simulink model "slb_gain"  (R2015b)
settings: Solver=FixedStepDiscrete  SolverMode=SingleTasking  StartTime=0.0  StopTime=10.0  RelTol=1e-3
PreLoadFcn:
  | A1 = 4
  | A2 = 10
  | A3 = 231
libraries: simulink x3
settings Model: Creator=amatsumo  LastModifiedBy=amatsumo
settings DataIOCC: SaveFormat=Array  SignalLoggingSaveFormat=ModelDataLogs  SaveOutput=off  SignalLogging=off  SaveTime=off
settings OptimizationCC: BlockReduction=off  ConditionallyExecuteInputs=off  DefaultParameterBehavior=Inlined  ExpressionDepthLimit=2147483647
settings DebuggingCC: AlgebraicLoopMsg=error  UnderspecifiedInitializationDetection=Classic  MergeDetectMultiDrivingBlocksExec=none  SolverPrmCheckMsg=warning  InheritedTsInSrcMsg=none  SingleTaskRateTransMsg=error  FcnCallInpInsideContextMsg=UseLocalSettings  StateNameClashWarn=warning
settings HardwareCC: ProdBitPerPointer=32  ProdLargestAtomicFloat=None  ProdIntDivRoundTo=Undefined  ProdEndianess=Unspecified  ProdWordSize=32  ProdHWDeviceType=ASIC/FPGA->ASIC/FPGA  ProdEqTarget=off
settings GRTTargetCC: GeneratePreprocessorConditionals=Disable all  CombineOutputUpdateFcns=off  GRTInterface=on
settings ConfigComp: CovModelRefEnable=Off  CovSFcnEnable=off

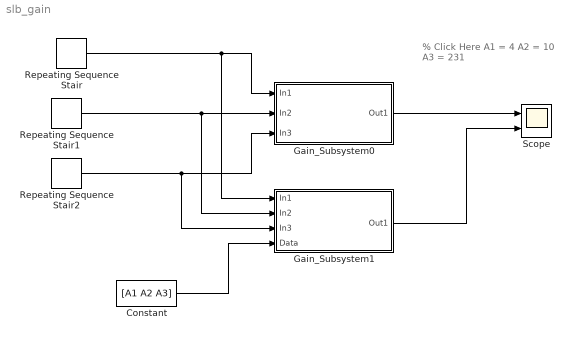
== system slb_gain ==
  note: % Click Here
      | A1 = 4
      | A2 = 10
      | A3 = 231
  Constant : Constant  Value=[A1 A2 A3]  OutDataTypeStr=fixdt(1,16,6)  SampleTime=-1
  Gain_Subsystem0 : Subsystem
  Gain_Subsystem1 : Subsystem
  Repeating Sequence Stair : simulink/Sources/Repeating Sequence Stair  OutValues=[3 1 4 2 1].'  tsamp=0.1  OutMin=[]  OutMax=[]  OutDataTypeStr=int8  OutputDataTypeScalingMode=int8  OutDataType=double  ConRadixGroup=Best Precision: Vector-wise  OutScaling=2^-12
  Repeating Sequence Stair1 : simulink/Sources/Repeating Sequence Stair  OutValues=[3 1 4 2 1].'  tsamp=0.1  OutMin=[]  OutMax=[]  OutDataTypeStr=int8  OutputDataTypeScalingMode=int8  OutDataType=double  ConRadixGroup=Best Precision: Vector-wise  OutScaling=2^-12
  Repeating Sequence Stair2 : simulink/Sources/Repeating Sequence Stair  OutValues=[3 1 4 2 1].'  tsamp=0.1  OutMin=[]  OutMax=[]  OutDataTypeStr=int8  OutputDataTypeScalingMode=int8  OutDataType=double  ConRadixGroup=Best Precision: Vector-wise  OutScaling=2^-12
  Scope : Scope  NumInputPorts=2
  wires:
  Repeating Sequence Stair/1 -> Gain_Subsystem0/1(In1), Gain_Subsystem1/1(In1)
  Repeating Sequence Stair1/1 -> Gain_Subsystem0/2(In2), Gain_Subsystem1/2(In2)
  Gain_Subsystem0/1(Out1) -> Scope/1
  Repeating Sequence Stair2/1 -> Gain_Subsystem0/3(In3), Gain_Subsystem1/3(In3)
  Gain_Subsystem1/1(Out1) -> Scope/2
  Constant/1 -> Gain_Subsystem1/4(Data)

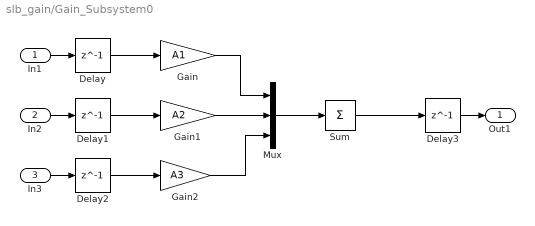
== system slb_gain/Gain_Subsystem0 ==
  In1 : Inport
  In2 : Inport  Port=2
  In3 : Inport  Port=3
  Delay : Delay  RequirementInfo="{}  %GIDa_6632c933_ccf5_4ee7_8d76_ef4c0c495654"  DelayLength=1
  Delay1 : Delay  RequirementInfo={} %GIDa_c975783b_ed1d_4928_ab74_9487ea49e7a0  DelayLength=1
  Delay2 : Delay  RequirementInfo={} %GIDa_a0fb7fe2_7995_4bc4_bc6b_c3fd8f13fd3e  DelayLength=1
  Delay3 : Delay  RequirementInfo={} %GIDa_bb9459df_f642_410c_997c_7de29e0468ab  DelayLength=1
  Gain : Gain  Gain=A1  ParamDataTypeStr=fixdt(1,16,8)  OutDataTypeStr=fixdt(1,16,5)
  Gain1 : Gain  Gain=A2  ParamDataTypeStr=fixdt(1,16,8)  OutDataTypeStr=fixdt(1,16,5)
  Gain2 : Gain  Gain=A3  ParamDataTypeStr=fixdt(1,16,4)  OutDataTypeStr=fixdt(1,16,5)
  Mux : Mux  Inputs=3
  Sum : Sum  Inputs=+
  Out1 : Outport
  wires:
  Delay/1 -> Gain/1
  Delay1/1 -> Gain1/1
  Delay2/1 -> Gain2/1
  Gain/1 -> Mux/1
  Gain1/1 -> Mux/2
  Gain2/1 -> Mux/3
  Mux/1 -> Sum/1
  In1/1 -> Delay/1
  In2/1 -> Delay1/1
  Delay3/1 -> Out1/1
  In3/1 -> Delay2/1
  Sum/1 -> Delay3/1

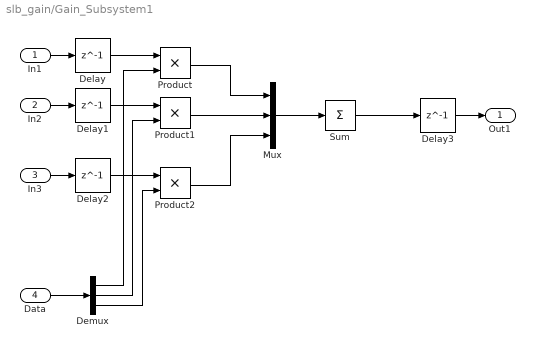
== system slb_gain/Gain_Subsystem1 ==
  In1 : Inport
  In2 : Inport  Port=2
  In3 : Inport  Port=3
  Data : Inport  Port=4
  Delay : Delay  RequirementInfo="{}  %GIDa_6632c933_ccf5_4ee7_8d76_ef4c0c495654"  DelayLength=1
  Delay1 : Delay  RequirementInfo={} %GIDa_48c29bca_111b_4f63_a60b_4d4a9bc347c1  DelayLength=1
  Delay2 : Delay  RequirementInfo={} %GIDa_6a9a2d78_2b77_479e_9eee_db7fc2816dbf  DelayLength=1
  Delay3 : Delay  RequirementInfo={} %GIDa_48743cef_953b_4e6e_b4f1_58dbb0f72e65  DelayLength=1
  Demux : Demux  Outputs=3
  Mux : Mux  Inputs=3
  Product : Product  OutDataTypeStr=fixdt(1,16,6)
  Product1 : Product  OutDataTypeStr=fixdt(1,16,6)
  Product2 : Product  OutDataTypeStr=fixdt(1,16,6)
  Sum : Sum  Inputs=+
  Out1 : Outport
  wires:
  Sum/1 -> Delay3/1
  In3/1 -> Delay2/1
  Delay3/1 -> Out1/1
  In2/1 -> Delay1/1
  In1/1 -> Delay/1
  Mux/1 -> Sum/1
  Product2/1 -> Mux/3
  Product1/1 -> Mux/2
  Product/1 -> Mux/1
  Delay2/1 -> Product2/1
  Delay1/1 -> Product1/1
  Delay/1 -> Product/1
  Data/1 -> Demux/1
  Demux/1 -> Product/2
  Demux/2 -> Product1/2
  Demux/3 -> Product2/2
